simulink model "MSE312_FinalModel"  (R2023a)
settings: Solver=ode5  StartTime=0.0  StopTime=inf  FixedStep=0.01  RelTol=1e-3  EnableMultiTasking=on
libraries: arduinolib x7, dspstat3 x2, eeGeneralControl x1, slpidlib x1, simulink x1, arduinosensorlib x1, RASPlib x1, robotcorelib x1
settings Model: ExtModeTrigDuration=2  Creator=mwa140  LastModifiedBy=abn2
settings OptimizationCC: EnhancedBackFolding=on  PassReuseOutputArgsAs=Individual arguments  ZeroExternalMemoryAtStartup=off  ZeroInternalMemoryAtStartup=off  MaxStackSize=64  OptimizeBlockOrder=speed  DifferentSizesBufferReuse=on  OptimizationCustomize=off  EfficientTunableParamExpr=on
settings DebuggingCC: ParameterTunabilityLossMsg=error
settings HardwareCC: ProdBitPerInt=16  ProdBitPerPointer=16  ProdBitPerSizeT=16  ProdBitPerPtrDiffT=16  ProdLargestAtomicFloat=None  ProdWordSize=8  ProdHWDeviceType=Atmel->AVR
settings SFSimCC: MATLABDynamicMemAlloc=off
settings RTWCC: Description=Embedded Coder  SystemTargetFile=ert.tlc  HardwareBoard=Arduino Mega 2560  TemplateMakefile=ert_default_tmf  Toolchain=Arduino AVR  BuildConfiguration=Faster Runs
settings CodeAppCC: ForceParamTrailComments=on  IgnoreCustomStorageClasses=off  OperatorAnnotations=on  SimulinkDataObjDesc=on  SFDataObjDesc=on  InsertBlockDesc=on
settings ERTTargetCC: SupportContinuousTime=on  SupportVariableSizeSignals=on  ExtModeTransport=3  ExtModeStaticAlloc=on  ExtModeAutomaticAllocSize=off  ExtModeStaticAllocSize=2048  ExtModeMexFile=ext_xcp  ExtModeIntrfLevel=Level2 - Open

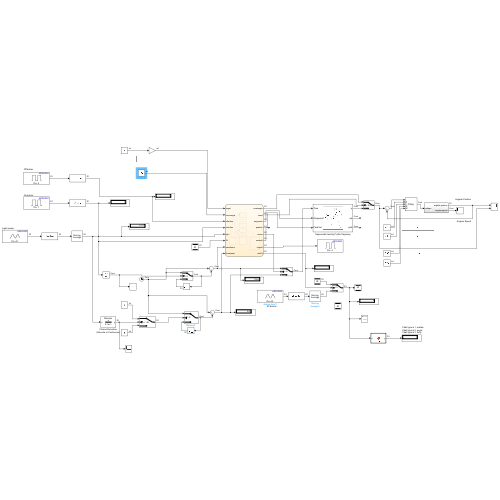
[thumbnail: Simulink's stored preview of the top-level diagram]
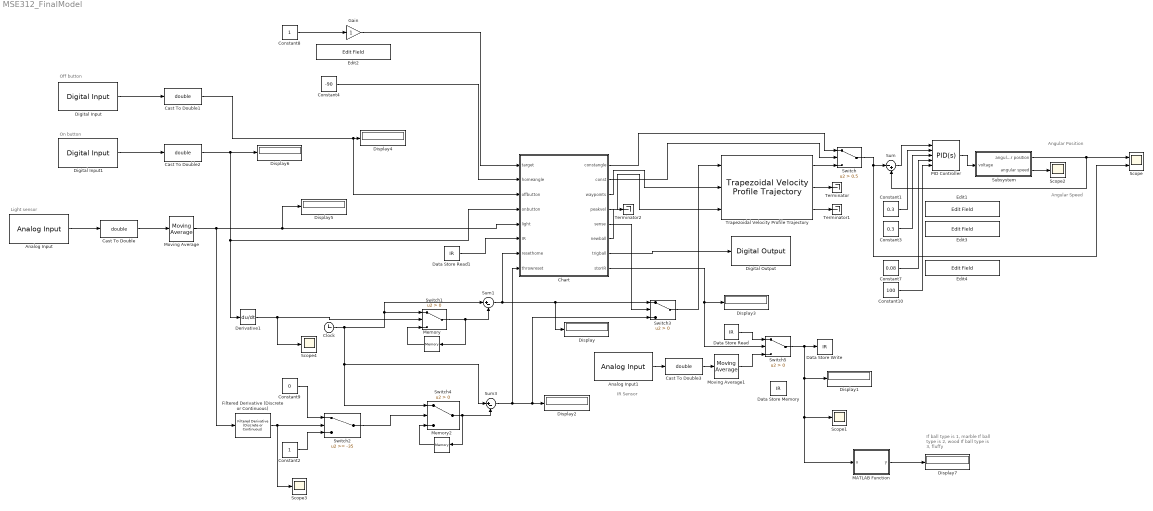
== system MSE312_FinalModel ==
  note: If ball type is 1, marble
      | If ball type is 2, wood
      | If ball type is 3, fluffy
  note: IR Sensor
  note: Light sensor
  note: On button
  note: Off button
  note: Angular Speed
  note: Angular Position
  Analog Input : arduinolib/Analog Input  pinNumber=1  ReadResultsOnly=off  ConversionTriggerSource=Software  ExternalTriggerType=uint32( 0 )  OutputDataType=uint16  EnableConversionCompleteNotify=off  EnableOuputStatus=off  SampleTime=0.01  blockPlatform=arduino
  Analog Input1 : arduinolib/Analog Input  pinNumber=0  ReadResultsOnly=off  ConversionTriggerSource=Software  ExternalTriggerType=uint32( 0 )  OutputDataType=uint16  EnableConversionCompleteNotify=off  EnableOuputStatus=off  SampleTime=0.01  blockPlatform=arduino
  Cast To Double{,1..3} (4 alike) : DataTypeConversion  OutDataTypeStr=double  SaturateOnIntegerOverflow=off  RndMeth=Floor
  Chart : Stateflow chart  TreatAsAtomicUnit=on
      settings: PortSchema="{\"entries\":[{\"content\":{\"sides\":[{\"content\":{\"connectorIds\":[\"In1\",\"In2\",\"In3\",\"In4\",\"In5\",\"In6\",\"In7\",\"In8\"]},\"type\":\"ConnectorPlacement.EquallySpacedRectSide\",\"uuid\":\"e8bfdbd1-893b-42e6-b43a-0b2b3f4c9105\"},{\"content\":{\"connectorIds\":[\"Out1\",\"Out2\",\"Out3\",\"Out6\",\"Out7\",\"Out8\",\"Out4\",\"Out5\"],\"side\":\"RIGHT\"},\"type\":\"ConnectorPlacement.EquallySpacedRectSide\",\"uuid\":\"8d111112-8bea-466f-bcfd-d9691d7f51af\"},{\"content\":{\"side\":\"TOP\"},\"type\":\"ConnectorPlacement.EquallySpacedRectSide\",\"uuid\":\"d1e1a004-9ff7-4ccf-879b-906870c8af02\"}]},\"type\":\"ConnectorPlacement.EquallySpacedConnector\",\"uuid\":\"434310ae-80c0-487c-93a4-84c043b4a7b8\"}],\"packageUris\":[\"http://schema.mathworks.com/mf0/Connector/R2020b\"],\"version\":\"1.0\"}"
  Clock : Clock
  Constant1 : Constant  Value=0.3
  Constant10 : Constant  Value=100
  Constant2 : Constant
  Constant3 : Constant  Value=0.3
  Constant4 : Constant  Value=-90
  Constant7 : Constant  Value=0.08
  Constant8 : Constant
  Constant9 : Constant  Value=0
  Data Store Memory : DataStoreMemory  DataStoreName=IR  WriteAfterWriteMsg=warning  ShowAdditionalParam=off
  Data Store Read : DataStoreRead  DataStoreName=IR  IndexOptions=Index vector (dialog)  Indices=1  OutputSizes=1
  Data Store Read1 : DataStoreRead  DataStoreName=IR  SampleTime=0.01  IndexOptions=Index vector (dialog)  Indices=1  OutputSizes=1
  Data Store Write : DataStoreWrite  DataStoreName=IR  IndexOptions=Index vector (dialog)  Indices=1  OutputSizes=1
  Derivative1 : Derivative
  Digital Input : arduinolib/Digital Input  pinNumber=6  mode=Default  Direction=input  SampleTime=0.01  blockPlatform=arduino
  Digital Input1 : arduinolib/Digital Input  pinNumber=7  mode=Default  Direction=input  SampleTime=0.01  blockPlatform=arduino
  Digital Output : arduinolib/Digital Output  pinNumber=4  Direction=output  blockPlatform=arduino
  Display{,1..7} (8 alike) : Display
  Edit{1..4} (4 alike) : EditField  LabelPosition=Hide  ShowInitialText=on  Alignment=Center
  Filtered Derivative (Discrete or Continuous) : eeGeneralControl/Filtered Derivative (Discrete or Continuous)  K=1  T=0.1  B=inf  A=-inf  minRatio=10  init_option=Inherited from block input  x0=0  Ts=-1
      settings: LibrarySourceBlock=|
      | ee_sl_lib/General Control/Filtered Derivative
      | (Discrete or Continuous)
  Gain : Gain
  MATLAB Function : MATLAB Function  TreatAsAtomicUnit=on
  Memory : Memory
  Memory2 : Memory
  Moving Average : dspstat3/Moving Average  Method=Sliding window  ForgettingFactorPort=off  SpecifyWindowLength=on  WindowLength=4  OverlapLength=3  AllowArbitraryInputLength=off  ForgettingFactor=0.9  SimulateUsing=Code generation
  Moving Average1 : dspstat3/Moving Average  Method=Sliding window  ForgettingFactorPort=off  SpecifyWindowLength=on  WindowLength=4  OverlapLength=3  AllowArbitraryInputLength=off  ForgettingFactor=0.9  SimulateUsing=Code generation
  PID Controller : slpidlib/PID Controller  Controller=PID  Form=Parallel  TimeDomain=Continuous-time  UseExternalTs=off  SampleTime=-1  IntegratorMethod=Forward Euler  FilterMethod=Forward Euler  ControllerParametersSource=external  P=.4  I=.4  UseKiTs=off  D=.075  N=100  UseFilter=on  TunerSelectOption=Transfer Function Based (PID Tuner App)  InitialConditionSource=internal  InitialConditionForIntegrator=0  InitialConditionForFilter=0  DifferentiatorICPrevScaledInput=0  ExternalReset=none  TrackingMode=off  Kt=1  LimitOutput=off  SatLimitsSource=internal  UpperSaturationLimit=inf  LowerSaturationLimit=-inf  LinearizeAsGain=on  AntiWindupMode=none  Kb=1  LimitIntegrator=off  UpperIntegratorSaturationLimit=inf  LowerIntegratorSaturationLimit=-inf  POutMin=[]  POutMax=[]  IOutMin=[]  IOutMax=[]  DOutMin=[]  DOutMax=[]  NOutMin=[]  NOutMax=[]  SumOutMin=[]  SumOutMax=[]  SaturationOutMin=[]  SaturationOutMax=[]  PParamMin=[]  PParamMax=[]  IParamMin=[]  IParamMax=[]  DParamMin=[]  DParamMax=[]  NParamMin=[]  NParamMax=[]  KbParamMin=[]  KbParamMax=[]  KtParamMin=[]  KtParamMax=[]  KbOutMin=[]  KbOutMax=[]  KtOutMin=[]  KtOutMax=[]  IntegratorOutMin=[]  IntegratorOutMax=[]  FilterOutMin=[]  FilterOutMax=[]  SumI1OutMin=[]  SumI1OutMax=[]  SumI2OutMin=[]  SumI2OutMax=[]  SumI3OutMin=[]  SumI3OutMax=[]  SumI4OutMin=[]  SumI4OutMax=[]  SumDOutMin=[]  SumDOutMax=[]  DifferentiatorOutMin=[]  DifferentiatorOutMax=[]  FilterDiffOutCoefMin=[]  FilterDiffOutCoefMax=[]  ReciprocalOutMin=[]  ReciprocalOutMax=[]  SumDenOutMin=[]  SumDenOutMax=[]  SumNumOutMin=[]  SumNumOutMax=[]  DivideOutMin=[]  DivideOutMax=[]  UdiffTsProdOutMin=[]  UdiffTsProdOutMax=[]  NTsProdOutMin=[]  NTsProdOutMax=[]  UintegralTsProdOutMin=[]  UintegralTsProdOutMax=[]  UngainTsProdOutMin=[]  UngainTsProdOutMax=[]  ClampingZeroOutDataTypeStr=Inherit: Inherit via back propagation  ClampingZeroOutMin=[]  ClampingZeroOutMax=[]  FilterDenConstantOutDataTypeStr=Inherit: Inherit via back propagation  FilterDenConstantOutMin=[]  FilterDenConstantOutMax=[]  PCopyOutDataTypeStr=Inherit: Inherit via back propagation  PCopyOutMin=[]  PCopyOutMax=[]  NCopyOutDataTypeStr=Inherit: Inherit via back propagation  NCopyOutMin=[]  NCopyOutMax=[]  IntegratorContinuousStateAttributes=''  IntegratorStateMustResolveToSignalObject=off  IntegratorRTWStateStorageClass=Auto  FilterContinuousStateAttributes=''  FilterStateMustResolveToSignalObject=off  FilterRTWStateStorageClass=Auto  ParallelPVariant=ExternalParameters  IdealPVariant=Disabled  IVariant=ExternalParameters  DVariant=ExternalParameters  IntegratorVariant=Continuous  SatVariant=Disabled  AWVariant=Passthrough  PCopyVariant=Disabled  TRVariant=Disabled  FdbkBlocksVariant=Forward  IdealPFdbkVariant=Disabled  SatFdbkVariant=Disabled  DerivativeFilterVariant=ContFilter  NVariant=ExternalParameters  NCopyVariant=Disabled  FilterICVariant=InternalICsFilter  IntegratorICVariant=InternalICs  ExternalResetVariant=Disabled  TRSumVariant=Passthrough  SumFdbkVariant=Disabled  SumVariant=Sum_PID  TsampFilterVariant=InternalTs  TsampNgainVariant=Passthrough  TsampIntegralVariant=Disabled_SignalSpec  ExternalSaturationOutDataTypeStr=Inherit: Same as second input
  Scope : Scope  NumInputPorts=2
  Scope{1..4} (4 alike) : Scope
  Subsystem : Subsystem
  Sum : Sum  Inputs=|-+
  Sum1 : Sum  Inputs=|+-
  Sum3 : Sum  Inputs=|+-
  Switch : Switch  Criteria=u2 > Threshold  Threshold=0.5  SaturateOnIntegerOverflow=off  InputSameDT=off
  Switch{1,3..5} (4 alike) : Switch  Criteria=u2 > Threshold  SaturateOnIntegerOverflow=off  InputSameDT=off
  Switch2 : Switch  Threshold=-35  SaturateOnIntegerOverflow=off  InputSameDT=off
  Terminator : Terminator
  Terminator1 : Terminator
  Terminator2 : Terminator
  Trapezoidal Velocity Profile Trajectory : robotcorelib/Trapezoidal Velocity Profile Trajectory  WaypointSource=External  Waypoints=[0,90,0]  NumParams=1  Parameter1=Peak Velocity  Parameter2=End Time  ParameterSource=External  PeakVelocity=[ 2; 2 ]  Acceleration=[ 1; 2 ]  EndTime=[ 1; 1 ]  AccelTime=[ 1; 2 ]  SimulateUsing=Interpreted execution
  wires:
  Subsystem/1(angular position) -> Sum/2, Scope/1
  Subsystem/2(angular speed) -> Scope2/1
  Sum/1 -> PID Controller/1
  PID Controller/1 -> Subsystem/1(voltage)
  Trapezoidal Velocity Profile Trajectory/2 -> Terminator/1
  Trapezoidal Velocity Profile Trajectory/3 -> Terminator1/1
  Chart/3(waypoints) -> Trapezoidal Velocity Profile Trajectory/2
  Chart/6(peakvel) -> Trapezoidal Velocity Profile Trajectory/3
  Trapezoidal Velocity Profile Trajectory/1 -> Switch/3
  Switch/1 -> Sum/1, Scope/2
  Chart/2(const) -> Switch/2
  Chart/1(constangle) -> Switch/1
  Clock/1 -> Sum1/1, Switch1/1, Switch4/1, Sum3/1
  Switch1/1 -> Sum1/2, Memory/1
  Sum1/1 -> Display/1, Switch3/1, Chart/7(resethome)
  Constant4/1 -> Chart/2(homeangle)
  Switch3/1 -> Trapezoidal Velocity Profile Trajectory/1
  Switch4/1 -> Sum3/2, Memory2/1
  Sum3/1 -> Switch3/3, Display2/1, Chart/8(throwreset)
  Chart/7(sense) -> Switch3/2
  Chart/8(newball) -> Terminator2/1
  Cast To Double/1 -> Moving Average/1
  Memory2/1 -> Switch4/3
  Constant8/1 -> Gain/1
  Gain/1 -> Chart/1(target)
  Analog Input/1 -> Cast To Double/1
  Moving Average/1 -> Filtered Derivative (Discrete or Continuous)/1, Display5/1, Chart/5(light)
  Switch2/1 -> Switch4/2
  Constant2/1 -> Switch2/3
  Constant9/1 -> Switch2/1
  Chart/4(trigball) -> Digital Output/1
  Digital Input/1 -> Cast To Double1/1
  Digital Input1/1 -> Cast To Double2/1
  Derivative1/1 -> Scope4/1, Switch1/2
  Memory/1 -> Switch1/3
  Data Store Read/1 -> Switch5/1
  Chart/5(storIR) -> Switch5/2, Display3/1
  Analog Input1/1 -> Cast To Double3/1
  Cast To Double3/1 -> Moving Average1/1
  Switch5/1 -> MATLAB Function/1(u), Scope1/1, Display1/1, Data Store Write/1
  Data Store Read1/1 -> Chart/6(IR)
  Filtered Derivative (Discrete or Continuous)/1 -> Scope3/1, Switch2/2
  Cast To Double1/1 -> Chart/3(offbutton), Display4/1
  Cast To Double2/1 -> Display6/1, Derivative1/1, Chart/4(onbutton)
  Moving Average1/1 -> Switch5/3
  Constant1/1 -> PID Controller/2
  Constant3/1 -> PID Controller/3
  Constant7/1 -> PID Controller/4
  Constant10/1 -> PID Controller/5
  MATLAB Function/1(y) -> Display7/1

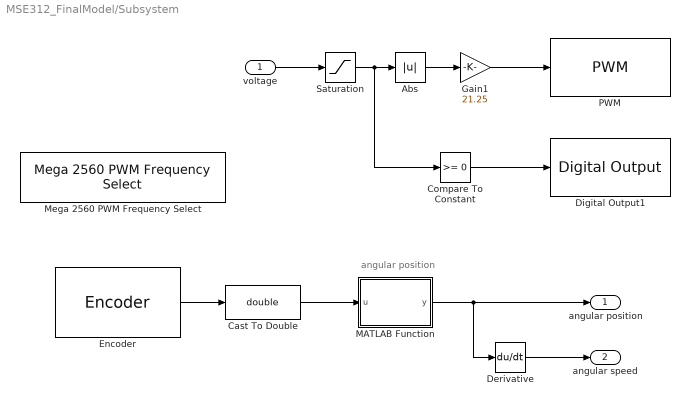
== system MSE312_FinalModel/Subsystem ==
  note: angular position
  voltage : Inport
  Abs : Abs  SaturateOnIntegerOverflow=off
  Cast To Double : DataTypeConversion  OutDataTypeStr=double  SaturateOnIntegerOverflow=off  RndMeth=Floor
  Compare To Constant : simulink/Logic and Bit Operations/Compare To Constant  relop=>=  const=0  OutDataTypeStr=boolean
  Derivative : Derivative  CoefficientInTFapproximation=0.01
  Digital Output1 : arduinolib/Digital Output  pinNumber=10  Direction=output  blockPlatform=arduino
  Encoder : arduinosensorlib/Encoder  InputA=2  InputB=3  Mode=No reset  SampleTime=0.01
  Gain1 : Gain  Gain=21.25
  MATLAB Function : MATLAB Function  TreatAsAtomicUnit=on
  Mega 2560 PWM Frequency Select : RASPlib/Mega 2560 PWM Frequency Select  Frequency=32KHz  Timer=2 - pins 9, 10
      settings: SourceProductName=Rensselaer Arduino Support Package
  PWM : arduinolib/PWM  pinNumber=9  frequencyType=Default  desiredFrequency=490.2  achievableFrequency=490.2
  Saturation : Saturate  UpperLimit=12  LowerLimit=-12
  angular position : Outport
  angular speed : Outport  Port=2
  wires:
  Cast To Double/1 -> MATLAB Function/1(u)
  MATLAB Function/1(y) -> Derivative/1, angular position/1
  Derivative/1 -> angular speed/1
  Saturation/1 -> Compare To Constant/1, Abs/1
  Gain1/1 -> PWM/1
  Abs/1 -> Gain1/1
  Compare To Constant/1 -> Digital Output1/1
  voltage/1 -> Saturation/1
  Encoder/1 -> Cast To Double/1

== matlab function MSE312_FinalModel/MATLAB Function ==
  data: u input; y output
function y = fcn(u)
if u<50
    y=1;
elseif u<130
    y=2;
else
    y=3;
end

== matlab function MSE312_FinalModel/Subsystem/MATLAB Function ==
  data: u input; y output
function y = fcn(u)

pos=360/(500*4*6.3);
%pause(1);

y = pos*u;

== stateflow chart MSE312_FinalModel/Chart ==
  state SwOff
    entry:
    waypoints=[0,0,0]
    constangle=0
    peakvel=0
    const=1
    sense=1
    newball=0
    storIR=0
    trigball=0
  state SwOn
    %entry:
    %waypoints=[0,-180,0]
    constangle=homeangle
  state Home
    during:
    %if resethome>15
    %waypoints=[0,0,0]
    %peakvel=0
    %end
  state Home2
    entry:
    newball=0
    storIR=1
    trigball=1
  state BallExisting
  state Wood
    entry:
    sense=0
    const=1
    trigball=0
    during:
    if throwreset>1
    constangle=homeangle+20;
    if throwreset>4
    constangle=homeangle-125
    if throwreset>7
    constangle=homeangle;
    peakvel=0; newball=1; trigball=0
    end
    end
    end
    exit:
    storIR=0
  state Marble
    entry:
    sense=0
    const=0
    trigball=0
    waypoints=[homeangle,homeangle+110,homeangle]
    peakvel=30
    during:
    if throwreset>10
    waypoints=[homeangle,homeangle, homeangle]
    peakvel=0; newball=1;trigball=0
    end
    exit:
    storIR=0;
  state Fluffy
    entry:
    sense=0
    const=1
    trigball=0
    if target==1.2
    constangle=homeangle-100;
    elseif target>=1.1
    constangle=homeangle-110;
    elseif target>=1
    constangle=homeangle-120
    end
    during:
    if throwreset>1
    constangle=homeangle;
    peakvel=0; newball=1; trigball=0
    end
    exit:
    storIR=0;
  (default) -> SwOff
  Wood -> SwOff [order 2] : [offbutton>0.5]
  BallExisting -> SwOff [order 4] : [offbutton>0.5]
  Home2 -> SwOff [order 1] : [offbutton>0.5]
  Home -> SwOff [order 1] : [offbutton>0.5]
  SwOn -> SwOff [order 1] : [offbutton>0.5]
  SwOff -> SwOn : [onbutton>0.5]
  SwOn -> Home [order 2]
  Home -> Home2 [order 2] : [peakvel==0]
  Wood -> Home2 [order 1] : [newball==1]
  Fluffy -> Home2 : [newball==1]
  Marble -> Home2 : [newball==1]
  Home2 -> BallExisting [order 2] : [light<5]
  BallExisting -> Wood [order 2] : [IR>=50 && IR<=130]
  BallExisting -> Marble [order 1] : [IR<50]
  BallExisting -> Fluffy [order 3] : [IR>130]
  data: target input; homeangle input; offbutton input; onbutton input; constangle output; const output; light input; IR input; waypoints output; trigball output; storIR output; peakvel output; resethome input; sense output; throwreset input; newball output
